simulink model "scars_model"  (R2019b)
settings: Solver=FixedStepAuto  StartTime=0.0  StopTime=300  FixedStep=0.01  MaxStep=1  MinStep=dT  RelTol=1e-3
model workspace (MAT data in the model file):
  actuators = 0
values from neighbouring files (symbols this model uses):
  decsec = decyear(2000,1,1,12,0,1) - decyear(2000,1,1,12,0,0)    [SCARSSetup.m]    (also in pwsat2_setup.m; pwsat2_tle.m; scars_setup.m)
  decstart = decyear(utc)    [SCARSSetup.m]    (also in pwsat2_setup.m; pwsat2_tle.m; scars_setup.m)
  forcesBody = [0 0 0]    [SCARSSetup.m]    (also in pwsat2_setup.m; scars_setup.m)
  initEuler = [0 0 0]    [SCARSSetup.m]    (also in pwsat2_setup.m; scars_setup.m)
  initMoments = [0 0 0]    [SCARSSetup.m]    (also in pwsat2_setup.m; scars_setup.m)
  momentsBody = [0 0 0]    [SCARSSetup.m]    (also in pwsat2_setup.m; scars_setup.m)
  refEuler = [0 0 1]    [SCARSSetup.m]    (also in pwsat2_setup.m = [0 deg2rad(45) deg2rad(45)]; scars_setup.m)
  refVel = [v_b(1) v_b(2) v_b(3)]    [SCARSSetup.m]    (also in pwsat2_setup.m; scars_setup.m)
undefined symbols (not defined in the file or in its folder): bb, Earth, gyro, rw, thruster, WGS84, WMM2000
libraries: scars_library x10, simulink_extras x2, aerolibgravity2 x2, simulink x1, aerolib6dof2 x1, sharedtransform x1, aerolibutil x1
settings Model: OrderedModelArguments=off  Creator=asmialek  LastModifiedBy=asmialek
settings DataIOCC: SaveFormat=Array  ReturnWorkspaceOutputsName=scars_out

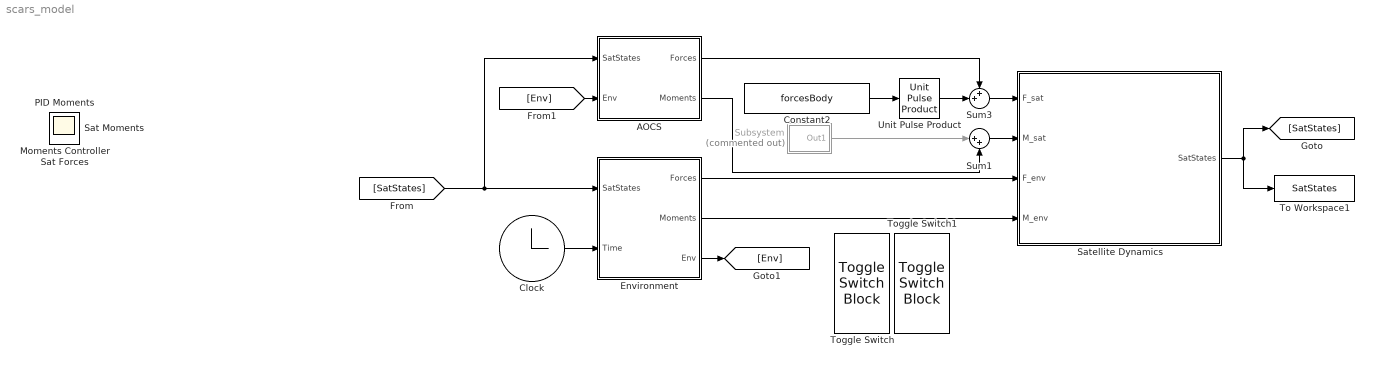
== system scars_model ==
  AOCS : Subsystem
  Clock : Clock
  Constant2 : Constant  Value=forcesBody
  Environment : Subsystem
  Satellite Dynamics : Subsystem
  Subsystem : Subsystem  Commented=on
  Sum1 : Sum  Inputs=|++
  Sum3 : Sum  Inputs=++|
  To Workspace1 : ToWorkspace  VariableName=SatStates  SaveFormat=Timeseries  SampleTime=-1
  Toggle Switch : ToggleSwitchBlock
      settings: Values={{'Off', 'On'}, [0 1]}
  Toggle Switch1 : ToggleSwitchBlock
      settings: Values={{'Off', 'On'}, [0 1]}
  Unit Pulse Product : scars_library/Unit Pulse Product  SystemSampleTime=-1  Latency=0  AutoFrameSizeCalculation=off
  Moments Controller : Scope
  PID Moments : Scope
  Sat Forces : Scope
  Sat Moments : Scope
  wires:
  Constant2/1 -> Unit Pulse Product/1
  Unit Pulse Product/1 -> Sum3/2
  Satellite Dynamics/1(SatStates) -> To Workspace1/1, [SatStates]
  [SatStates] -> AOCS/1(SatStates), Environment/1(SatStates)
  Environment/1(Forces) -> Satellite Dynamics/3(F_env)
  Environment/2(Moments) -> Satellite Dynamics/4(M_env)
  Sum3/1 -> Satellite Dynamics/1(F_sat)
  Subsystem/1(Out1) -> Sum1/1
  Sum1/1 -> Satellite Dynamics/2(M_sat)
  Clock/1 -> Environment/2(Time)
  Environment/3(Env) -> [Env]
  [Env] -> AOCS/2(Env)
  AOCS/1(Forces) -> Sum3/1
  AOCS/2(Moments) -> Sum1/2

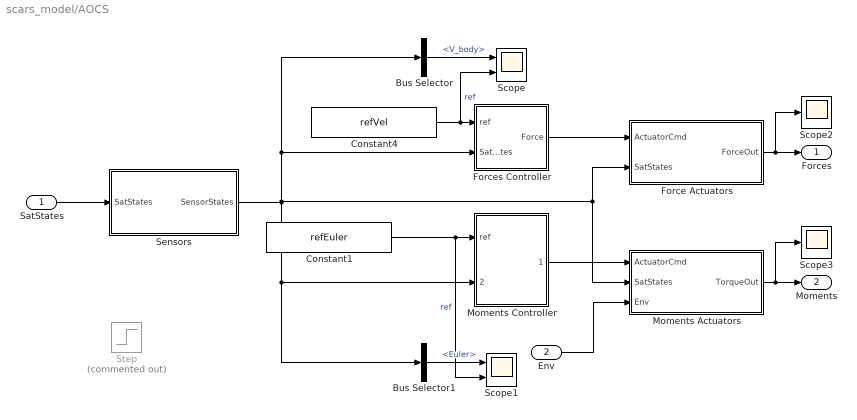
== system scars_model/AOCS ==
  SatStates : Inport
  Env : Inport  Port=2
  Bus Selector : BusSelector  OutputSignals=V_body
  Bus Selector1 : BusSelector  OutputSignals=Euler
  Constant1 : Constant  Value=refEuler
  Constant4 : Constant  Value=refVel
  Force Actuators : Subsystem
  Forces Controller : Subsystem
  Moments Actuators : Subsystem
  Moments Controller : Subsystem
  Scope : Scope  NumInputPorts=2
  Scope1 : Scope  NumInputPorts=2
  Scope2 : Scope
  Scope3 : Scope
  Sensors : Subsystem
  Step : Step  Commented=on  Time=3  After=refEuler  SampleTime=0
  Forces : Outport
  Moments : Outport  Port=2
  wires:
  Force Actuators/1(ForceOut) -> Scope2/1, Forces/1
  SatStates/1 -> Sensors/1(SatStates)
  Constant4/1 -> Scope/2, Forces Controller/1(ref)  "ref"
  Forces Controller/1(Force) -> Force Actuators/1(ActuatorCmd)
  Constant1/1 -> Scope1/2, Moments Controller/1(ref)  "ref"
  Bus Selector/1 -> Scope/1  "<V_body>"
  Bus Selector1/1 -> Scope1/1  "<Euler>"
  Moments Actuators/1(TorqueOut) -> Scope3/1, Moments/1
  Sensors/1(SensorStates) -> Bus Selector1/1, Moments Controller/2(SatStates), Moments Actuators/2(SatStates), Force Actuators/2(SatStates), Bus Selector/1, Forces Controller/2(SatStates)
  Env/1 -> Moments Actuators/3(Env)
  Moments Controller/1(Torque) -> Moments Actuators/1(ActuatorCmd)

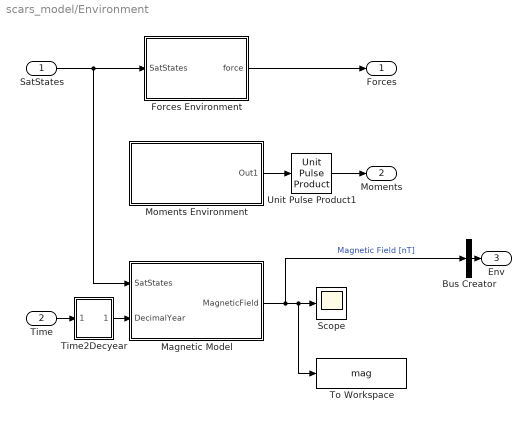
== system scars_model/Environment ==
  SatStates : Inport
  Time : Inport  Port=2
  Bus Creator : BusCreator  Inputs=1
  Forces Environment : Subsystem
  Magnetic Model : Subsystem
  Moments Environment : Subsystem
  Scope : Scope
  Time2Decyear : Subsystem
  To Workspace : ToWorkspace  VariableName=mag  SampleTime=-1
  Unit Pulse Product1 : scars_library/Unit Pulse Product  SystemSampleTime=-1  Latency=0  AutoFrameSizeCalculation=off
  Forces : Outport
  Moments : Outport  Port=2
  Env : Outport  Port=3
  wires:
  Moments Environment/1(Out1) -> Unit Pulse Product1/1
  SatStates/1 -> Magnetic Model/1(SatStates), Forces Environment/1(SatStates)
  Forces Environment/1(force) -> Forces/1
  Unit Pulse Product1/1 -> Moments/1
  Time/1 -> Time2Decyear/1(" ")
  Time2Decyear/1("  ") -> Magnetic Model/2(DecimalYear)
  Magnetic Model/1(MagneticField) -> Bus Creator/1, To Workspace/1, Scope/1  "Magnetic Field [nT]"
  Bus Creator/1 -> Env/1

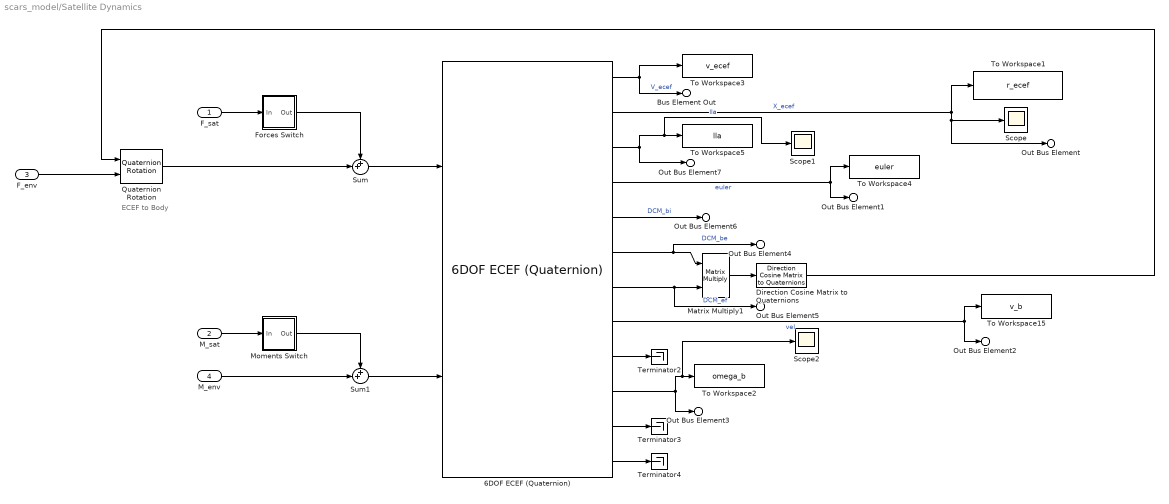
== system scars_model/Satellite Dynamics ==
  note: ECEF to Body
  F_sat : Inport
  M_sat : Inport  Port=2
  F_env : Inport  Port=3
  M_env : Inport  Port=4
  6DOF ECEF (Quaternion) : aerolib6dof2/6DOF ECEF (Quaternion)  units=Metric (MKS)  mtype=Fixed  xg_0=r_lla  Vm_0=v_b  eul_0=deg2rad(initEuler)  pm_0=[0 0 0]  mass_0=1.0  mass_e=0.5  mass_f=2.0  inertia=eye(3)  inertia_e=eye(3)  inertia_f=2*eye(3)  vre_flag=on  abi_flag=off  ptype=Earth (WGS84)  R=6378137  F=1/298.257223563  w_E=7292115e-11  angle_in=Internal  LG0=0  quat_statename=''  pm_statename=''  Vm_statename=''  posECEF_statename=''  posECI_statename=''  LG_statename=''  mass_statename=''
      settings: SourceProductName=Aerospace Blockset  SourceProductBaseCode=AE
  Direction Cosine Matrix to Quaternions : sharedtransform/Direction Cosine Matrix  to Quaternions  aMode=0  action=None  tolerance=eps(2)
      settings: SourceProductName=Aerospace Blockset  SourceProductBaseCode=AE
  Forces Switch : Subsystem
  Matrix Multiply1 : Product  Multiplication=Matrix(*)
  Moments Switch : Subsystem
  Quaternion Rotation : aerolibutil/Quaternion Rotation
  Scope : Scope
  Scope1 : Scope
  Scope2 : Scope
  Sum : Sum  Inputs=++|
  Sum1 : Sum  Inputs=++|
  Terminator2 : Terminator
  Terminator3 : Terminator
  Terminator4 : Terminator
  To Workspace1 : ToWorkspace  VariableName=r_ecef  SampleTime=-1
  To Workspace15 : ToWorkspace  VariableName=v_b  SampleTime=-1
      settings: Save2DSignal=2-D array (concatenate along first dimension)
  To Workspace2 : ToWorkspace  VariableName=omega_b  SampleTime=-1
      settings: Save2DSignal=2-D array (concatenate along first dimension)
  To Workspace3 : ToWorkspace  VariableName=v_ecef  SampleTime=-1
      settings: Save2DSignal=2-D array (concatenate along first dimension)
  To Workspace4 : ToWorkspace  VariableName=euler  SampleTime=-1
      settings: Save2DSignal=2-D array (concatenate along first dimension)
  To Workspace5 : ToWorkspace  VariableName=lla  SampleTime=-1
      settings: Save2DSignal=2-D array (concatenate along first dimension)
  Bus Element Out : Outport  PortName=SatStates  Element=V_ecef
  Out Bus Element : Outport  PortName=SatStates  Element=X_ecef
  Out Bus Element1 : Outport  PortName=SatStates  Element=Euler
  Out Bus Element2 : Outport  PortName=SatStates  Element=V_body
  Out Bus Element3 : Outport  PortName=SatStates  Element=Omega_body
  Out Bus Element6 : Outport  PortName=SatStates  Element=ECI2Body
  Out Bus Element4 : Outport  PortName=SatStates  Element=NED2Body
  Out Bus Element5 : Outport  PortName=SatStates  Element=ECEF2NED
  Out Bus Element7 : Outport  PortName=SatStates  Element=lla
  wires:
  6DOF ECEF (Quaternion)/1 -> To Workspace3/1, Bus Element Out/1  "V_ecef"
  6DOF ECEF (Quaternion)/8 -> Out Bus Element2/1, To Workspace15/1  "vel"
  6DOF ECEF (Quaternion)/2 -> Scope/1, Out Bus Element/1, To Workspace1/1  "X_ecef"
  6DOF ECEF (Quaternion)/6 -> Out Bus Element4/1, Matrix Multiply1/1  "DCM_be"
  Sum/1 -> 6DOF ECEF (Quaternion)/1
  6DOF ECEF (Quaternion)/7 -> Out Bus Element5/1, Matrix Multiply1/2  "DCM_ef"
  6DOF ECEF (Quaternion)/4 -> Out Bus Element1/1, To Workspace4/1  "euler"
  6DOF ECEF (Quaternion)/10 -> Scope2/1, To Workspace2/1, Out Bus Element3/1
  M_env/1 -> Sum1/2
  Sum1/1 -> 6DOF ECEF (Quaternion)/2
  Matrix Multiply1/1 -> Direction Cosine Matrix to Quaternions/1
  F_sat/1 -> Forces Switch/1(In)
  Quaternion Rotation/1 -> Sum/2
  F_env/1 -> Quaternion Rotation/2
  Direction Cosine Matrix to Quaternions/1 -> Quaternion Rotation/1
  Forces Switch/1(Out) -> Sum/1
  M_sat/1 -> Moments Switch/1(In)
  Moments Switch/1(Out) -> Sum1/1
  6DOF ECEF (Quaternion)/5 -> Out Bus Element6/1  "DCM_bi"
  6DOF ECEF (Quaternion)/9 -> Terminator2/1
  6DOF ECEF (Quaternion)/11 -> Terminator3/1
  6DOF ECEF (Quaternion)/12 -> Terminator4/1
  6DOF ECEF (Quaternion)/3 -> Out Bus Element7/1, Scope1/1, To Workspace5/1  "lla"

== system scars_model/Subsystem ==
  Constant1 : Constant  Value=momentsBody
  Constant2 : Constant  Value=momentsBody
  Gain : Gain  Gain=-1
  Sum : Sum  Inputs=|++
  Unit Pulse Product1 : scars_library/Unit Pulse Product  SystemSampleTime=-1  Latency=0  AutoFrameSizeCalculation=off
  Unit Pulse Product2 : scars_library/Unit Pulse Product  SystemSampleTime=-1  Latency=0  AutoFrameSizeCalculation=off
  Out1 : Outport
  wires:
  Constant1/1 -> Unit Pulse Product1/1
  Unit Pulse Product1/1 -> Sum/1
  Sum/1 -> Out1/1
  Constant2/1 -> Unit Pulse Product2/1
  Gain/1 -> Sum/2
  Unit Pulse Product2/1 -> Gain/1

== system scars_model/AOCS/Force Actuators ==
  ActuatorCmd : Inport
  Bus Element In : Inport  Port=2  PortName=SatStates  Element=V_ecef
  Actuator Choice : Constant  Value=2
  Combo Box : ComboBox  LabelPosition=Hide  SelectedLabel=Thrusters
      settings: Values={{'Perfect Actuators', 'Thrusters', 'idontknowyet', 'No Actuators'}, [1 2 3 4]}
  Constant : Constant  Value=[0 0 0]
  Constant1 : Constant  Value=[0 0 0]
  Directional Thrusters : scars_library/Perfect Actuators  SystemSampleTime=-1  Latency=0  AutoFrameSizeCalculation=off
  Multiport Switch : MultiPortSwitch  Inputs=4  DiagnosticForDefault=Warning
  Perfect Actuators : scars_library/Perfect Actuators  SystemSampleTime=-1  Latency=0  AutoFrameSizeCalculation=off
  Terminator : Terminator
  ForceOut : Outport
  wires:
  Perfect Actuators/1 -> Multiport Switch/2
  Constant/1 -> Multiport Switch/5
  Actuator Choice/1 -> Multiport Switch/1
  Directional Thrusters/1 -> Multiport Switch/3
  ActuatorCmd/1 -> Directional Thrusters/1, Perfect Actuators/1
  Multiport Switch/1 -> ForceOut/1
  Constant1/1 -> Multiport Switch/4
  Bus Element In/1 -> Terminator/1

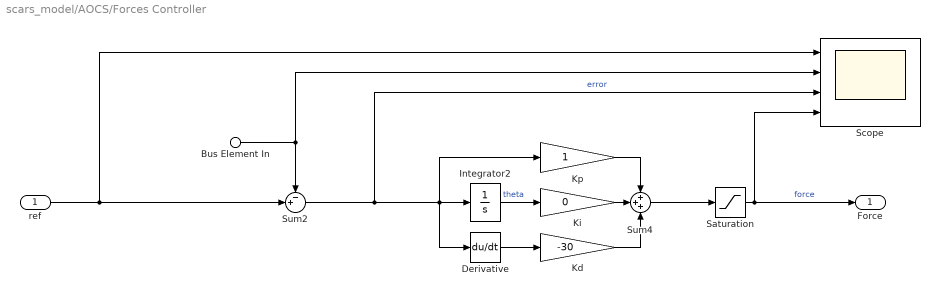
== system scars_model/AOCS/Forces Controller ==
  ref : Inport
  Bus Element In : Inport  Port=2  PortName=SatStates  Element=V_body
  Derivative : Derivative
  Integrator2 : Integrator
  Kd : Gain  Gain=-30
  Ki : Gain  Gain=0
  Kp : Gain
  Saturation : Saturate  UpperLimit=3  LowerLimit=-3
  Scope : Scope  NumInputPorts=4
  Sum2 : Sum  Inputs=-+|
  Sum4 : Sum  Inputs=+++
  Force : Outport
  wires:
  Saturation/1 -> Force/1, Scope/4  "force"
  ref/1 -> Sum2/2, Scope/1
  Sum4/1 -> Saturation/1
  Bus Element In/1 -> Sum2/1, Scope/2
  Kd/1 -> Sum4/3
  Kp/1 -> Sum4/1
  Sum2/1 -> Kp/1, Derivative/1, Integrator2/1, Scope/3  "error"
  Ki/1 -> Sum4/2
  Derivative/1 -> Kd/1
  Integrator2/1 -> Ki/1  "theta"

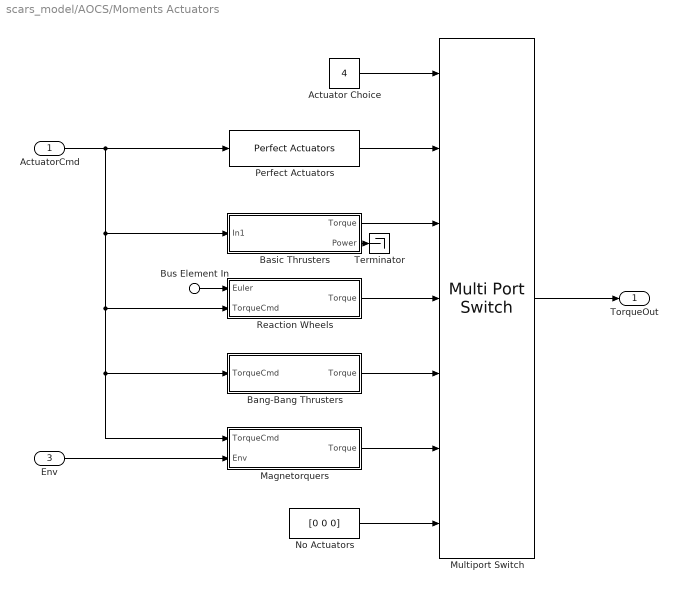
== system scars_model/AOCS/Moments Actuators ==
  ActuatorCmd : Inport
  Bus Element In : Inport  Port=2  PortName=SatStates  Element=Euler
  Env : Inport  Port=3
  Actuator Choice : Constant  Value=4
  Bang-Bang Thrusters : Subsystem
  Basic Thrusters : Subsystem
  Magnetorquers : Subsystem
  Multiport Switch : MultiPortSwitch  Inputs=6  DiagnosticForDefault=Warning
  No Actuators : Constant  Value=[0 0 0]
  Perfect Actuators : scars_library/Perfect Actuators  SystemSampleTime=-1  Latency=0  AutoFrameSizeCalculation=off
  Reaction Wheels : Subsystem
  Terminator : Terminator
  TorqueOut : Outport
  wires:
  Perfect Actuators/1 -> Multiport Switch/2
  Bang-Bang Thrusters/1(Torque) -> Multiport Switch/5
  Actuator Choice/1 -> Multiport Switch/1
  Reaction Wheels/1(Torque) -> Multiport Switch/4
  Multiport Switch/1 -> TorqueOut/1
  ActuatorCmd/1 -> Basic Thrusters/1(In1), Magnetorquers/1(TorqueCmd), Bang-Bang Thrusters/1(TorqueCmd), Reaction Wheels/2(TorqueCmd), Perfect Actuators/1
  Bus Element In/1 -> Reaction Wheels/1(Euler)
  Basic Thrusters/1(Torque) -> Multiport Switch/3
  No Actuators/1 -> Multiport Switch/7
  Magnetorquers/1(Torque) -> Multiport Switch/6
  Basic Thrusters/2(Power) -> Terminator/1
  Env/1 -> Magnetorquers/2(Env)

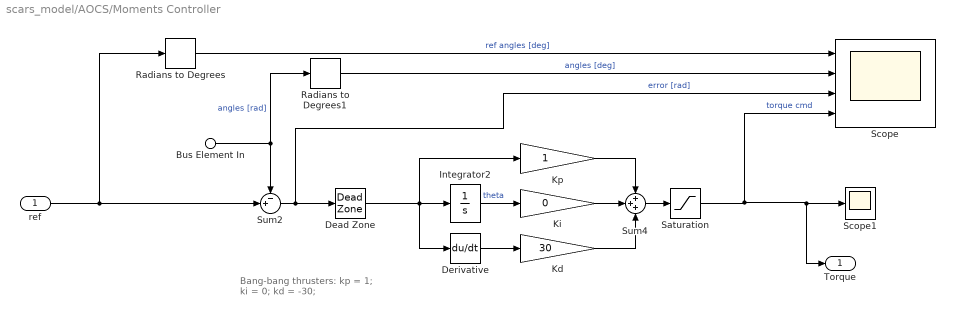
== system scars_model/AOCS/Moments Controller ==
  note: Bang-bang thrusters:
      | kp = 1;
      | ki = 0;
      | kd = -30;
  ref : Inport
  Bus Element In : Inport  Port=2  PortName=SatStates  Element=Euler
  Dead Zone : DeadZone  LowerValue=-1e-3  UpperValue=1e-3  SaturateOnIntegerOverflow=on
  Derivative : Derivative
  Integrator2 : Integrator
  Kd : Gain  Gain=30
  Ki : Gain  Gain=0
  Kp : Gain
  Radians to Degrees : simulink_extras/Transformations/Radians to Degrees
  Radians to Degrees1 : simulink_extras/Transformations/Radians to Degrees
  Saturation : Saturate  UpperLimit=3  LowerLimit=-3
  Scope : Scope  NumInputPorts=4
  Scope1 : Scope
  Sum2 : Sum  Inputs=-+|
  Sum4 : Sum  Inputs=+++
  Torque : Outport
  wires:
  Saturation/1 -> Torque/1, Scope1/1, Scope/4  "torque cmd"
  ref/1 -> Sum2/2, Radians to Degrees/1
  Bus Element In/1 -> Sum2/1, Radians to Degrees1/1  "angles [rad]"
  Radians to Degrees/1 -> Scope/1  "ref angles [deg]"
  Radians to Degrees1/1 -> Scope/2  "angles [deg]"
  Kd/1 -> Sum4/3
  Sum4/1 -> Saturation/1
  Kp/1 -> Sum4/1
  Sum2/1 -> Scope/3, Dead Zone/1  "error [rad]"
  Ki/1 -> Sum4/2
  Derivative/1 -> Kd/1
  Integrator2/1 -> Ki/1  "theta"
  Dead Zone/1 -> Kp/1, Derivative/1, Integrator2/1

== system scars_model/AOCS/Sensors ==
  SatStates : Inport
  Bus Creator : BusCreator  Inputs=9
  Bus Selector : BusSelector  OutputSignals=V_ecef,X_ecef,Euler,V_body,Omega_body,lla,ECI2Body,ECEF2NED,NED2Body
  Gyros : Subsystem  Commented=through
  SensorStates : Outport
  wires:
  SatStates/1 -> Bus Selector/1
  Bus Creator/1 -> SensorStates/1
  Bus Selector/7 -> Bus Creator/7  "<ECI2Body>"
  Bus Selector/8 -> Bus Creator/8  "<ECEF2NED>"
  Bus Selector/9 -> Bus Creator/9  "<NED2Body>"
  Bus Selector/6 -> Bus Creator/6  "<lla>"
  Bus Selector/5 -> Gyros/1(In1)  "<Omega_body>"
  Bus Selector/4 -> Bus Creator/4  "<V_body>"
  Bus Selector/3 -> Bus Creator/3  "<Euler>"
  Bus Selector/1 -> Bus Creator/1  "<V_ecef>"
  Gyros/1(Out1) -> Bus Creator/5  "Omega_body"
  Bus Selector/2 -> Bus Creator/2  "<X_ecef>"

== system scars_model/Environment/Forces Environment ==
  Bus Element In : Inport  PortName=SatStates  Element=X_ecef
  Spherical Harmonic Gravity Model1 : aerolibgravity2/Spherical Harmonic Gravity Model  units=Metric (MKS)  degree=120  action=Warning  ptype=EGM2008  datafile='aerogmm2b.mat'
      settings: SourceProductName=Aerospace Blockset  SourceProductBaseCode=AE
  To Workspace13 : ToWorkspace  VariableName=g  SampleTime=-1
  force : Outport
  wires:
  Spherical Harmonic Gravity Model1/1 -> force/1, To Workspace13/1
  Bus Element In/1 -> Spherical Harmonic Gravity Model1/1

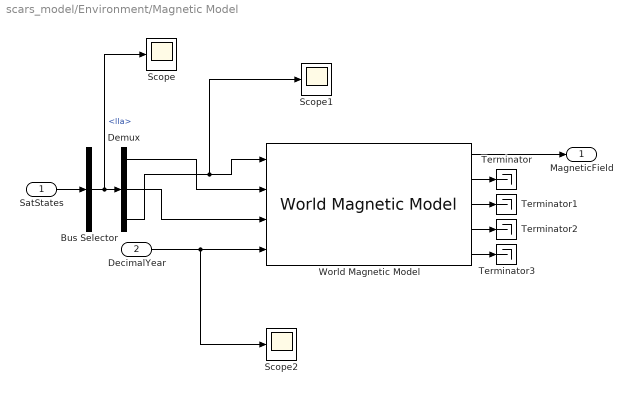
== system scars_model/Environment/Magnetic Model ==
  SatStates : Inport
  DecimalYear : Inport  Port=2
  Bus Selector : BusSelector  OutputSignals=lla
  Demux : Demux  Outputs=3
  Scope : Scope
  Scope1 : Scope
  Scope2 : Scope
  Terminator{,1..3} (4 alike) : Terminator
  World Magnetic Model : aerolibgravity2/World Magnetic Model  model=WMM2000 (2000-2005)  customFile='WMM2015v2.COF'  units=Metric (MKS)  time_in=on  month=January  day=1  year=2015  action=Error  h_out=on  dec_out=on  inc_out=on  ti_out=on
      settings: SourceProductName=Aerospace Blockset  SourceProductBaseCode=AE
  MagneticField : Outport
  wires:
  SatStates/1 -> Bus Selector/1
  DecimalYear/1 -> Scope2/1, World Magnetic Model/4
  World Magnetic Model/1 -> MagneticField/1
  World Magnetic Model/2 -> Terminator/1
  World Magnetic Model/5 -> Terminator3/1
  World Magnetic Model/3 -> Terminator1/1
  World Magnetic Model/4 -> Terminator2/1
  Bus Selector/1 -> Scope/1, Demux/1  "<lla>"
  Demux/1 -> World Magnetic Model/2
  Demux/2 -> World Magnetic Model/3
  Demux/3 -> Scope1/1, World Magnetic Model/1

== system scars_model/Environment/Moments Environment ==
  Constant : Constant  Value=initMoments
  Out1 : Outport
  wires:
  Constant/1 -> Out1/1

== system scars_model/Environment/Time2Decyear ==
  " " : Inport
  Decsec : Gain  Gain=decsec
  Initial Decyear : Constant  Value=decstart
  Sum : Sum  Inputs=|++
  "  " : Outport
  wires:
  Initial Decyear/1 -> Sum/1
  " "/1 -> Decsec/1
  Decsec/1 -> Sum/2
  Sum/1 -> "  "/1

== system scars_model/Satellite Dynamics/Forces Switch ==
  In : Inport
  Constant1 : Constant  Value=[0 0 0]
  Forces : Constant  Value=0
  Switch : Switch  Criteria=u2 > Threshold
  Out : Outport
  wires:
  Constant1/1 -> Switch/3
  Forces/1 -> Switch/2
  Switch/1 -> Out/1
  In/1 -> Switch/1

== system scars_model/Satellite Dynamics/Moments Switch ==
  In : Inport
  Constant1 : Constant  Value=[0 0 0]
  Moments : Constant
  Switch : Switch  Criteria=u2 > Threshold
  Out : Outport
  wires:
  In/1 -> Switch/1
  Constant1/1 -> Switch/3
  Switch/1 -> Out/1
  Moments/1 -> Switch/2

== system scars_model/AOCS/Moments Actuators/Bang-Bang Thrusters ==
  TorqueCmd : Inport
  Demux : Demux  Outputs=3
  Gain : Gain  Gain=-1
  Mux : Mux  Inputs=3
  Thruster Pitch : Subsystem
  Thruster Roll : Subsystem
  Thruster Yaw : Subsystem
  Torque : Outport  VectorParamsAs1DForOutWhenUnconnected=off
  wires:
  Thruster Roll/1(Torque Out) -> Mux/1
  Thruster Pitch/1(Torque Out) -> Mux/2
  Thruster Yaw/1(Torque Out) -> Mux/3
  TorqueCmd/1 -> Demux/1
  Demux/2 -> Thruster Pitch/1(Torque)
  Demux/1 -> Thruster Roll/1(Torque)
  Demux/3 -> Thruster Yaw/1(Torque)
  Mux/1 -> Gain/1
  Gain/1 -> Torque/1

== system scars_model/AOCS/Moments Actuators/Basic Thrusters ==
  In1 : Inport
  Basic Thrusters : scars_library/Basic Thrusters  SystemSampleTime=-1  Latency=0  AutoFrameSizeCalculation=off
  Basic Thrusters1 : scars_library/Basic Thrusters  SystemSampleTime=-1  Latency=0  AutoFrameSizeCalculation=off
  Basic Thrusters2 : scars_library/Basic Thrusters  SystemSampleTime=-1  Latency=0  AutoFrameSizeCalculation=off
  Constant : Constant  Value=thruster.distance
  Demux : Demux  Outputs=3
  Mux : Mux  Inputs=3
  Product : Product
  Sum : Sum  Inputs=+++
  Torque : Outport
  Power : Outport  Port=2
  wires:
  In1/1 -> Demux/1
  Demux/1 -> Basic Thrusters/1
  Basic Thrusters/1 -> Mux/1
  Demux/2 -> Basic Thrusters1/1
  Basic Thrusters1/1 -> Mux/2
  Basic Thrusters2/1 -> Mux/3
  Demux/3 -> Basic Thrusters2/1
  Basic Thrusters/2 -> Sum/1
  Basic Thrusters2/2 -> Sum/3
  Basic Thrusters1/2 -> Sum/2
  Constant/1 -> Product/2
  Mux/1 -> Product/1
  Product/1 -> Torque/1
  Sum/1 -> Power/1

== system scars_model/AOCS/Moments Actuators/Magnetorquers ==
  TorqueCmd : Inport
  Env : Inport  Port=2
  Terminator : Terminator
  Torque : Outport
  wires:
  TorqueCmd/1 -> Torque/1
  Env/1 -> Terminator/1

== system scars_model/AOCS/Moments Actuators/Reaction Wheels ==
  Euler : Inport
  TorqueCmd : Inport  Port=2
  Demux : Demux  Outputs=3
  Demux2 : Demux  Outputs=3
  Mux : Mux  Inputs=3
  Reaction Wheel Pitch : Subsystem
  Reaction Wheel Roll : Subsystem
  Reaction Wheel Yaw : Subsystem
  Torque : Outport  VectorParamsAs1DForOutWhenUnconnected=off
  wires:
  Mux/1 -> Torque/1
  Demux/1 -> Reaction Wheel Roll/2(Torque)
  Reaction Wheel Roll/1(Torque Out) -> Mux/1
  Demux2/1 -> Reaction Wheel Roll/1(Rate)
  Demux2/2 -> Reaction Wheel Pitch/1(Rate)
  Demux/2 -> Reaction Wheel Pitch/2(Torque)
  Demux2/3 -> Reaction Wheel Yaw/1(Rate)
  Demux/3 -> Reaction Wheel Yaw/2(Torque)
  Reaction Wheel Pitch/1(Torque Out) -> Mux/2
  Reaction Wheel Yaw/1(Torque Out) -> Mux/3
  Euler/1 -> Demux2/1
  TorqueCmd/1 -> Demux/1

== system scars_model/AOCS/Sensors/Gyros ==
  note: noise_power  = [0.1]
      | sample_time = 0.1
  note: wn = 1000*2*pi; % natural frequency [not in Hz, but can be transferred] dynamics rad/s
      | w = 12.5*2*pi; % cutoff frequency [Hz*2pi = deg/s] LPF rad/s
      | zeta = sqrt(2)/2; % damping ratio
      | z = zeta; %?
  In1 : Inport
  Add : Sum
  Add1 : Sum
  Band-Limited White Noise : simulink/Sources/Band-Limited White Noise  Cov=[gyro.noise_power]  Ts=gyro.sample_time  seed=[23341]
  Constant : Constant  Value=gyro.bias
  Rate Transition1 : RateTransition  OutPortSampleTime=gyro.rate
  Transfer Fcn : TransferFcn  Numerator=[gyro.wn^2]  Denominator=[1 2*gyro.zeta*gyro.wn gyro.wn^2]
  Transfer Fcn1 : TransferFcn  Numerator=[gyro.w^2]  Denominator=[1 2*gyro.z*gyro.w gyro.w^2]
  saturation of counts : Saturate  UpperLimit=gyro.max  LowerLimit=gyro.min
  scale factor dps 2 counts : Gain
  Out1 : Outport
  wires:
  Transfer Fcn/1 -> Add/1
  Constant/1 -> Add/2
  Add/1 -> Add1/1
  Band-Limited White Noise/1 -> Add1/2
  Add1/1 -> scale factor dps 2 counts/1
  scale factor dps 2 counts/1 -> saturation of counts/1
  saturation of counts/1 -> Transfer Fcn1/1
  Transfer Fcn1/1 -> Rate Transition1/1
  In1/1 -> Transfer Fcn/1
  Rate Transition1/1 -> Out1/1

== system scars_model/AOCS/Moments Actuators/Bang-Bang Thrusters/Thruster Pitch ==
  Torque : Inport
  Gain2 : Gain  Gain=-1
  Relay1 : Relay  OnSwitchValue=bb.a1  OffSwitchValue=bb.a0  OnOutputValue=bb.thrust
  Relay2 : Relay  OnSwitchValue=bb.a1  OffSwitchValue=bb.a0  OnOutputValue=-bb.thrust
  Scope1 : Scope  NumInputPorts=5
  Sum1 : Sum  Inputs=-|-
  Sum2 : Sum  Inputs=+|+
  Torque Out : Outport
  wires:
  Sum1/1 -> Torque Out/1  "M"
  Relay2/1 -> Scope1/3, Sum2/2
  Sum2/1 -> Scope1/5, Sum1/1
  Gain2/1 -> Scope1/2, Relay2/1
  Relay1/1 -> Scope1/4, Sum2/1
  Torque/1 -> Scope1/1, Relay1/1, Gain2/1  "pd"

== system scars_model/AOCS/Moments Actuators/Bang-Bang Thrusters/Thruster Roll ==
  Torque : Inport
  Gain2 : Gain  Gain=-1
  Relay1 : Relay  OnSwitchValue=bb.a1  OffSwitchValue=bb.a0  OnOutputValue=bb.thrust
  Relay2 : Relay  OnSwitchValue=bb.a1  OffSwitchValue=bb.a0  OnOutputValue=-bb.thrust
  Scope1 : Scope  NumInputPorts=5
  Sum1 : Sum  Inputs=-|-
  Sum2 : Sum  Inputs=+|+
  Torque Out : Outport
  wires:
  Sum1/1 -> Torque Out/1  "M"
  Relay2/1 -> Scope1/3, Sum2/2
  Sum2/1 -> Scope1/5, Sum1/1
  Gain2/1 -> Scope1/2, Relay2/1
  Relay1/1 -> Scope1/4, Sum2/1
  Torque/1 -> Scope1/1, Relay1/1, Gain2/1  "pd"

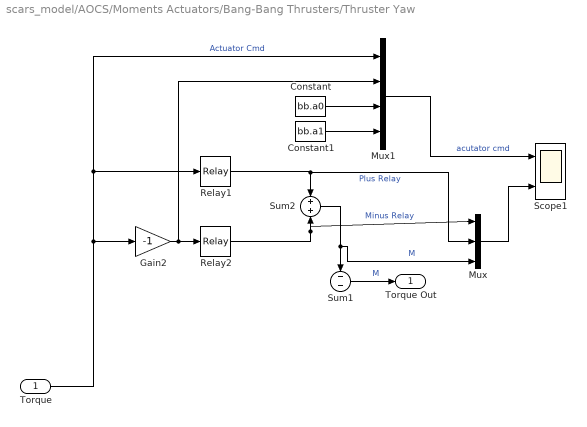
== system scars_model/AOCS/Moments Actuators/Bang-Bang Thrusters/Thruster Yaw ==
  Torque : Inport
  Constant : Constant  Value=bb.a0
  Constant1 : Constant  Value=bb.a1
  Gain2 : Gain  Gain=-1
  Mux : Mux  Inputs=3
  Mux1 : Mux
  Relay1 : Relay  OnSwitchValue=bb.a1  OffSwitchValue=bb.a0  OnOutputValue=bb.thrust
  Relay2 : Relay  OnSwitchValue=bb.a1  OffSwitchValue=bb.a0  OnOutputValue=-bb.thrust
  Scope1 : Scope  NumInputPorts=2
  Sum1 : Sum  Inputs=-|-
  Sum2 : Sum  Inputs=+|+
  Torque Out : Outport
  wires:
  Sum1/1 -> Torque Out/1  "M"
  Relay2/1 -> Mux/1, Sum2/2  "Minus Relay"
  Sum2/1 -> Mux/3, Sum1/1  "M"
  Gain2/1 -> Mux1/2, Relay2/1
  Relay1/1 -> Mux/2, Sum2/1  "Plus Relay"
  Torque/1 -> Relay1/1, Mux1/1, Gain2/1  "Actuator Cmd"
  Mux1/1 -> Scope1/1  "acutator cmd"
  Mux/1 -> Scope1/2
  Constant/1 -> Mux1/3
  Constant1/1 -> Mux1/4

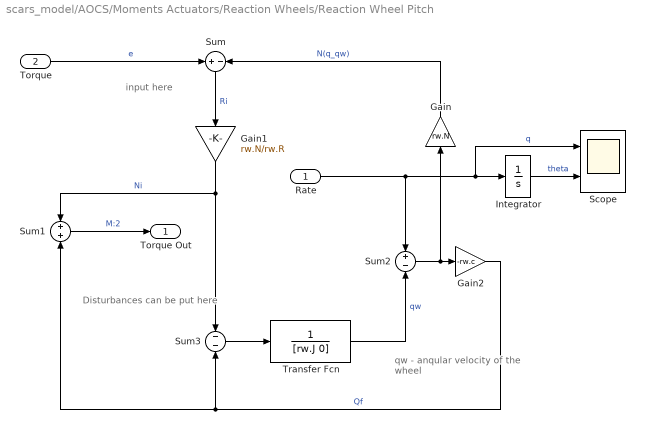
== system scars_model/AOCS/Moments Actuators/Reaction Wheels/Reaction Wheel Pitch ==
  note: qw - anqular velocity
      |  of the wheel
  note: input here
  note: Disturbances can
      | be put here
  Rate : Inport
  Torque : Inport  Port=2
  Gain : Gain  Gain=rw.N
  Gain1 : Gain  Gain=rw.N/rw.R
  Gain2 : Gain  Gain=-rw.c
  Integrator : Integrator
  Scope : Scope  NumInputPorts=2
  Sum : Sum  Inputs=+|-
  Sum1 : Sum  Inputs=+|+
  Sum2 : Sum  Inputs=+|-
  Sum3 : Sum  Inputs=-|-
  Transfer Fcn : TransferFcn  Denominator=[rw.J 0]
  Torque Out : Outport
  wires:
  Gain2/1 -> Sum1/2, Sum3/2  "Qf"
  Gain1/1 -> Sum1/1, Sum3/1  "Ni"
  Integrator/1 -> Scope/2  "theta"
  Sum3/1 -> Transfer Fcn/1
  Torque/1 -> Sum/1  "e"
  Sum1/1 -> Torque Out/1  "M:2"
  Gain/1 -> Sum/2  "N(q_qw)"
  Rate/1 -> Sum2/1, Integrator/1, Scope/1  "q"
  Sum2/1 -> Gain/1, Gain2/1
  Sum/1 -> Gain1/1  "Ri"
  Transfer Fcn/1 -> Sum2/2  "qw"

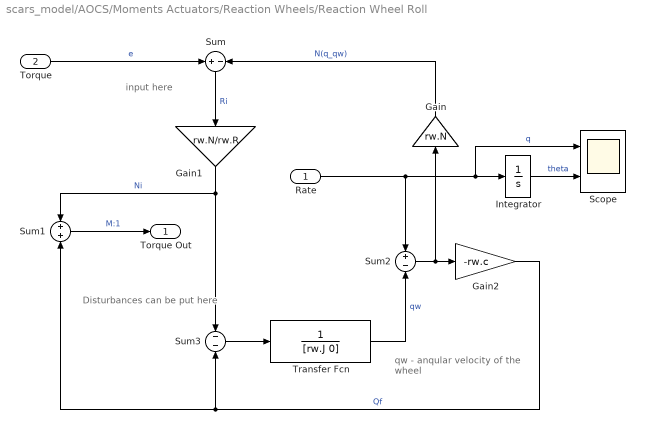
== system scars_model/AOCS/Moments Actuators/Reaction Wheels/Reaction Wheel Roll ==
  note: Disturbances can
      | be put here
  note: input here
  note: qw - anqular velocity
      |  of the wheel
  Rate : Inport
  Torque : Inport  Port=2
  Gain : Gain  Gain=rw.N
  Gain1 : Gain  Gain=rw.N/rw.R
  Gain2 : Gain  Gain=-rw.c
  Integrator : Integrator
  Scope : Scope  NumInputPorts=2
  Sum : Sum  Inputs=+|-
  Sum1 : Sum  Inputs=+|+
  Sum2 : Sum  Inputs=+|-
  Sum3 : Sum  Inputs=-|-
  Transfer Fcn : TransferFcn  Denominator=[rw.J 0]
  Torque Out : Outport
  wires:
  Gain1/1 -> Sum1/1, Sum3/1  "Ni"
  Torque/1 -> Sum/1  "e"
  Sum3/1 -> Transfer Fcn/1
  Sum/1 -> Gain1/1  "Ri"
  Integrator/1 -> Scope/2  "theta"
  Transfer Fcn/1 -> Sum2/2  "qw"
  Gain2/1 -> Sum1/2, Sum3/2  "Qf"
  Sum1/1 -> Torque Out/1  "M:1"
  Sum2/1 -> Gain2/1, Gain/1
  Gain/1 -> Sum/2  "N(q_qw)"
  Rate/1 -> Sum2/1, Integrator/1, Scope/1  "q"

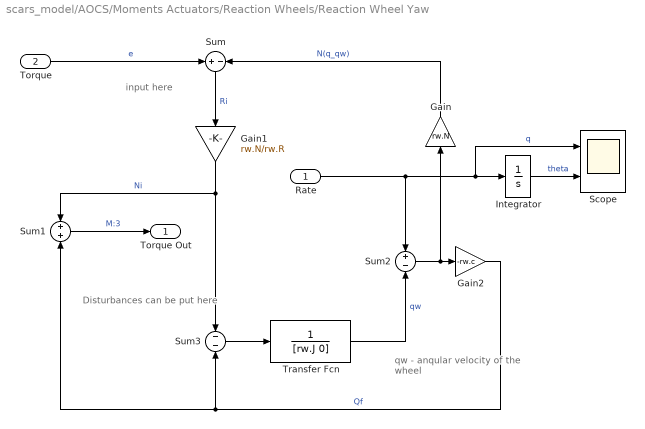
== system scars_model/AOCS/Moments Actuators/Reaction Wheels/Reaction Wheel Yaw ==
  note: qw - anqular velocity
      |  of the wheel
  note: input here
  note: Disturbances can
      | be put here
  Rate : Inport
  Torque : Inport  Port=2
  Gain : Gain  Gain=rw.N
  Gain1 : Gain  Gain=rw.N/rw.R
  Gain2 : Gain  Gain=-rw.c
  Integrator : Integrator
  Scope : Scope  NumInputPorts=2
  Sum : Sum  Inputs=+|-
  Sum1 : Sum  Inputs=+|+
  Sum2 : Sum  Inputs=+|-
  Sum3 : Sum  Inputs=-|-
  Transfer Fcn : TransferFcn  Denominator=[rw.J 0]
  Torque Out : Outport
  wires:
  Gain2/1 -> Sum1/2, Sum3/2  "Qf"
  Gain1/1 -> Sum1/1, Sum3/1  "Ni"
  Integrator/1 -> Scope/2  "theta"
  Sum3/1 -> Transfer Fcn/1
  Torque/1 -> Sum/1  "e"
  Sum1/1 -> Torque Out/1  "M:3"
  Gain/1 -> Sum/2  "N(q_qw)"
  Rate/1 -> Sum2/1, Integrator/1, Scope/1  "q"
  Sum2/1 -> Gain/1, Gain2/1
  Sum/1 -> Gain1/1  "Ri"
  Transfer Fcn/1 -> Sum2/2  "qw"
